simulink model "Tractive_Motor_Ring_Single_Motor"  (R2020a)
settings: Solver=FixedStepDiscrete  StartTime=0.0  StopTime=10.0  FixedStep=Ts  RelTol=1e-3  EnableMultiTasking=on
PostLoadFcn:
  | , if any(exist('dsrtsu_mdlpostloadfcn', 'file') ~= 0), dsrtsu_mdlpostloadfcn('Execute', bdroot); end,
InitFcn:
  | , if any(exist('rtifpga_mdlclblib', 'file') ~= 0), rtifpga_mdlclblib('Init', bdroot); end,
undefined symbols (not defined in the file): DiscIntNeverNeededParam, magnitude, TMR
libraries: simulink x3
settings Model: DSRTSU_INTERNAL_RTI_VER=560  DSRTSU_INTERNAL_RTI_TYPE=rti1401  RTICANMMDATA=struct('GeneralSetupData',struct('modelroot','C:\Users\harjo\Git\MACFormulaGit\MicroAutobox\rings\Tractive_Motor_Ring\Tractive_Motor_Ring_Single_Motor','generalsettings',struct('filesettings',struct('destfolder',struct('Name','RTICANMM_FILES','Check',1),'buildfolder',struct('Name','.','Check',1),'AbsDestfolder',struct('Name','C:\Users\harjo\Git\MACFormulaGit\MicroAutobox\rings\Tractive_Motor_Ring\Tractive_Motor_Ring_Single_Motor\RTICANMM_FILES'),'AbsBuildfolder',struct('Name','C:\Users\harjo\Git\MACFormulaGit\MicroAutobox\rings\Tractive_Motor_Ring\Tractive_Motor_Ring_Single_Motor'))),'options',struct('addpaths',1,'rmpaths',1,'addtrcexclusion',true,'cannavigator',struct('checkmonitoring',0),'show_usrtrc',0,'use_usrtrc',0),'advanced',struct('options',ones(1,100)),'MPSetup',{{}},'RTI',struct('Type','RTI1401','Ver','7.14','Date','02-May-2020'),'modelname','Tractive_Motor_Ring_Single_Motor','block','Tractive_Motor_Ring_Single_Motor'))  DSRTSU_INTERNAL_RTIFPGA=160  Creator=Harjot  LastModifiedBy=Harjot
settings DebuggingCC: SFUnexpectedBacktrackingDiag=warning  SFNoUnconditionalDefaultTransitionDiag=warning  SFExecutionAtInitializationDiag=none  ArithmeticOperatorsInVariantConditions=warning
settings HardwareCC: ProdBitPerPointer=32  ProdBitPerSizeT=32  ProdBitPerPtrDiffT=32  ProdLargestAtomicInteger=Integer  ProdEndianess=BigEndian  ProdWordSize=32  ProdHWDeviceType=Custom Processor->Custom  TargetIntDivRoundTo=Zero  TargetEndianess=BigEndian  TargetHWDeviceType=Custom Processor->Custom
settings SFSimCC: SimUseLocalCustomCode=off  MATLABDynamicMemAlloc=off  CustomCodeUndefinedFunction=UseInterfaceOnly
settings RTWCC: Description=dSPACE DS1401 Hardware Platform  SystemTargetFile=rti1401.tlc  MakeCommand=make_rti  TemplateMakefile=rti1401.tmf  RTWUseLocalCustomCode=off
settings CodeAppCC: StateflowObjectComments=on
settings STFCustomTargetCC: UtilityFuncGeneration=Shared location  ParMdlRefBuildCompliant=on  SystemTargetFile=rti1401.tlc
settings GRTTargetCC: TargetLangStandard=C89/C90 (ANSI)  UtilityFuncGeneration=Shared location  CompOptLevelCompliant=off  ConcurrentExecutionCompliant=off  CombineOutputUpdateFcns=off  MatFileLogging=off  CPPClassGenCompliant=off  UseToolchainInfoCompliant=off
settings ConfigComp: CovMetricSettings=dw  CovHtmlReporting=on  CovSaveCumulativeToWorkspaceVar=on  CovSaveSingleToWorkspaceVar=on  CovExternalEMLEnable=off

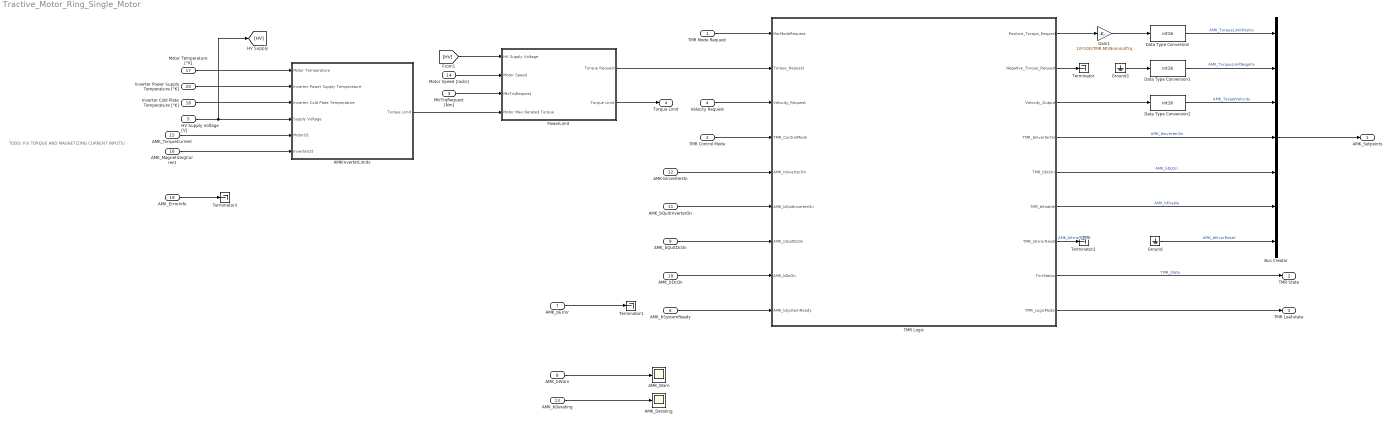
== system Tractive_Motor_Ring_Single_Motor ==
  note: TODO: FIX TORQUE AND MAGNETIZING CURRENT INPUTS!
  TMR Mode Request : Inport
  TMR Control Mode : Inport  Port=2
  MtrTrqRequest [Nm] : Inport  Port=3
  Velocity Request : Inport  Port=4
  HV Supply Voltage [V] : Inport  Port=5
  AMK_bSystemReady : Inport  Port=6  OutDataTypeStr=boolean  Interpolate=off  LockScale=on
  AMK_bError : Inport  Port=7  OutDataTypeStr=boolean  Interpolate=off  LockScale=on
  AMK_bWarn : Inport  Port=8  OutDataTypeStr=boolean  Interpolate=off
  AMK_bQuitDcOn : Inport  Port=9  OutDataTypeStr=boolean  Interpolate=off  LockScale=on
  AMK_bDcOn : Inport  Port=10  OutDataTypeStr=boolean  Interpolate=off  LockScale=on
  AMK_bQuitInverterOn : Inport  Port=11  OutDataTypeStr=boolean  LockScale=on
  AMK-bInverterOn : Inport  Port=12  OutDataTypeStr=boolean  Interpolate=off  LockScale=on
  AMK_bDerating : Inport  Port=13  OutDataTypeStr=boolean  Interpolate=off
  Motor Speed [rad/s] : Inport  Port=14
  AMK_TorqueCurrent : Inport  Port=15
  AMK_MagnetizingCurrent : Inport  Port=16
  Motor Temperature [°K] : Inport  Port=17  OutDataTypeStr=double
  Inverter Cold Plate Temperature [°K] : Inport  Port=18  OutDataTypeStr=double
  AMK_ErrorInfo : Inport  Port=19  OutDataTypeStr=double
  Inverter Power Supply Temperature [°K] : Inport  Port=20  OutDataTypeStr=double
  AMKInverterLimits : Subsystem
  AMK_Derating : Scope
  AMK_Warn : Scope
  Bus Creator : BusCreator  Inputs=7  OutDataTypeStr=Bus: AmkSetpoints  NonVirtualBus=on
      settings: InheritFromInputs=off
  Data Type Conversion : DataTypeConversion  OutDataTypeStr=int16
  Data Type Conversion1 : DataTypeConversion  OutDataTypeStr=int16
  Data Type Conversion2 : DataTypeConversion  OutDataTypeStr=int16
  Gain1 : Gain  Gain=10*100/TMR.MtrNominalTrq
  Ground : Ground
  Ground1 : Ground
  PowerLimit : Subsystem
  TMR Logic : Stateflow chart  TreatAsAtomicUnit=on
  Terminator{,1..3} (4 alike) : Terminator
  AMK_Setpoints : Outport  OutDataTypeStr=Bus: AmkSetpoints  VectorParamsAs1DForOutWhenUnconnected=off
  TMR State : Outport  Port=2  VectorParamsAs1DForOutWhenUnconnected=off
  TMR Leaf-state : Outport  Port=3  VectorParamsAs1DForOutWhenUnconnected=off
  Torque Limit : Outport  Port=4  VectorParamsAs1DForOutWhenUnconnected=off
  wires:
  TMR Logic/4(TMR_bInverterOn) -> Bus Creator/4  "AMK_bInverterOn"
  TMR Logic/6(TMR_bEnable) -> Bus Creator/6  "AMK_bEnable"
  TMR Logic/5(TMR_bDcOn) -> Bus Creator/5  "AMK_bDcOn"
  AMK_ErrorInfo/1 -> Terminator3/1
  AMK_bDerating/1 -> AMK_Derating/1
  AMK_bWarn/1 -> AMK_Warn/1
  Velocity Request/1 -> TMR Logic/3(Velocity_Request)
  AMK_bSystemReady/1 -> TMR Logic/9(AMK_bSystemReady)
  AMK_bQuitInverterOn/1 -> TMR Logic/6(AMK_bQuitInverterOn)
  Bus Creator/1 -> AMK_Setpoints/1
  TMR Logic/1(Positive_Torque_Request) -> Gain1/1
  TMR Control Mode/1 -> TMR Logic/4(TMR_ControlMode)
  TMR Logic/9(TMR_LogicMode) -> TMR Leaf-state/1
  Ground/1 -> Bus Creator/7  "AMK_bErrorReset"
  AMK_bQuitDcOn/1 -> TMR Logic/7(AMK_bQuitDcOn)
  AMK-bInverterOn/1 -> TMR Logic/5(AMK_bInverterOn)
  AMK_bDcOn/1 -> TMR Logic/8(AMK_bDcOn)
  TMR Logic/8(TmrStatus) -> TMR State/1  "TMR_State"
  TMR Mode Request/1 -> TMR Logic/1(MsrModeRequest)
  Data Type Conversion/1 -> Bus Creator/1  "AMK_TorqueLimitPositiv"
  Data Type Conversion1/1 -> Bus Creator/2  "AMK_TorqueLimitNegativ"
  Data Type Conversion2/1 -> Bus Creator/3  "AMK_TargetVelocity"
  TMR Logic/3(Velocity_Output) -> Data Type Conversion2/1
  Gain1/1 -> Data Type Conversion/1
  Ground1/1 -> Data Type Conversion1/1
  TMR Logic/2(Negative_Torque_Request) -> Terminator/1
  AMK_bError/1 -> Terminator1/1
  TMR Logic/7(TMR_bErrorReset) -> Terminator2/1  "AMK_bErrorReset"
  AMKInverterLimits/1(Torque Limit) -> PowerLimit/4(Motor Max Derated Torque)
  AMK_MagnetizingCurrent/1 -> AMKInverterLimits/6(InverterI2t)
  AMK_TorqueCurrent/1 -> AMKInverterLimits/5(MotorI2t)
  [HV] -> PowerLimit/1(HV Supply Voltage)
  HV Supply Voltage [V]/1 -> [HV], AMKInverterLimits/4(Supply Voltage)
  Inverter Cold Plate Temperature [°K]/1 -> AMKInverterLimits/3(Inverter Cold Plate Temperature)
  Inverter Power Supply Temperature [°K]/1 -> AMKInverterLimits/2(Inverter Power Supply Temperature)
  Motor Temperature [°K]/1 -> AMKInverterLimits/1(Motor Temperature)
  MtrTrqRequest [Nm]/1 -> PowerLimit/3(MtrTrqRequest)
  PowerLimit/1(Torque Request) -> TMR Logic/2(Torque_Request)
  PowerLimit/2(Torque Limit) -> Torque Limit/1
  Motor Speed [rad/s]/1 -> PowerLimit/2(Motor Speed)

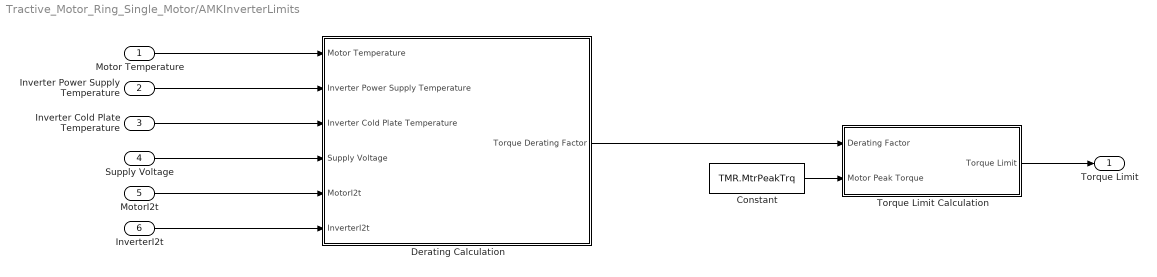
== system Tractive_Motor_Ring_Single_Motor/AMKInverterLimits ==
  Motor Temperature : Inport
  Inverter Power Supply Temperature : Inport  Port=2
  Inverter Cold Plate Temperature : Inport  Port=3
  Supply Voltage : Inport  Port=4
  MotorI2t : Inport  Port=5
  InverterI2t : Inport  Port=6
  Constant : Constant  Value=TMR.MtrPeakTrq
  Derating Calculation : Subsystem
  Torque Limit Calculation : Subsystem
  Torque Limit : Outport  VectorParamsAs1DForOutWhenUnconnected=off
  wires:
  Torque Limit Calculation/1(Torque Limit) -> Torque Limit/1
  InverterI2t/1 -> Derating Calculation/6(InverterI2t)
  Inverter Power Supply Temperature/1 -> Derating Calculation/2(Inverter Power Supply Temperature)
  Constant/1 -> Torque Limit Calculation/2(Motor Peak Torque)
  Motor Temperature/1 -> Derating Calculation/1(Motor Temperature)
  Derating Calculation/1(Torque Derating Factor) -> Torque Limit Calculation/1(Derating Factor)
  Inverter Cold Plate Temperature/1 -> Derating Calculation/3(Inverter Cold Plate Temperature)
  MotorI2t/1 -> Derating Calculation/5(MotorI2t)
  Supply Voltage/1 -> Derating Calculation/4(Supply Voltage)

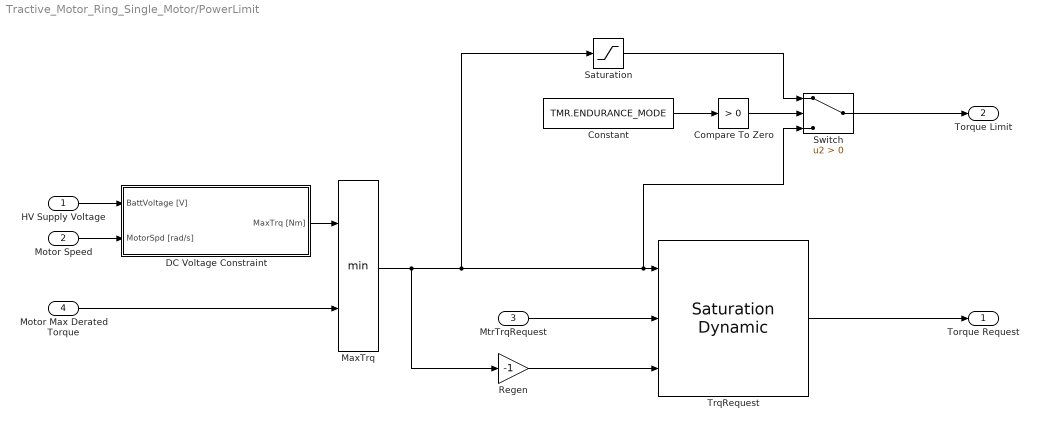
== system Tractive_Motor_Ring_Single_Motor/PowerLimit ==
  HV Supply Voltage : Inport
  Motor Speed : Inport  Port=2
  MtrTrqRequest : Inport  Port=3
  Motor Max Derated Torque : Inport  Port=4
  Compare To Zero : simulink/Logic and Bit Operations/Compare To Zero  relop=>  OutDataTypeStr=boolean
  Constant : Constant  Value=TMR.ENDURANCE_MODE
  DC Voltage Constraint : Subsystem
  MaxTrq : MinMax  Inputs=2
  Regen : Gain  Gain=-1
  Saturation : Saturate  UpperLimit=TMR.MtrNominalTrq  LowerLimit=0
  Switch : Switch  Criteria=u2 > Threshold
  TrqRequest : simulink/Discontinuities/Saturation Dynamic  OutMin=[]  OutMax=[]  OutDataTypeStr=Inherit: Same as second input  OutDataType=fixdt(1, 16)  OutScaling=2^-10  DoSatur=off
  Torque Request : Outport  VectorParamsAs1DForOutWhenUnconnected=off
  Torque Limit : Outport  Port=2  VectorParamsAs1DForOutWhenUnconnected=off
  wires:
  Saturation/1 -> Switch/1
  Switch/1 -> Torque Limit/1
  Compare To Zero/1 -> Switch/2
  Constant/1 -> Compare To Zero/1
  Regen/1 -> TrqRequest/3
  HV Supply Voltage/1 -> DC Voltage Constraint/1(BattVoltage [V])
  DC Voltage Constraint/1(MaxTrq [Nm]) -> MaxTrq/1
  MaxTrq/1 -> TrqRequest/1, Switch/3, Saturation/1, Regen/1
  Motor Speed/1 -> DC Voltage Constraint/2(MotorSpd [rad/s])
  TrqRequest/1 -> Torque Request/1
  Motor Max Derated Torque/1 -> MaxTrq/2
  MtrTrqRequest/1 -> TrqRequest/2

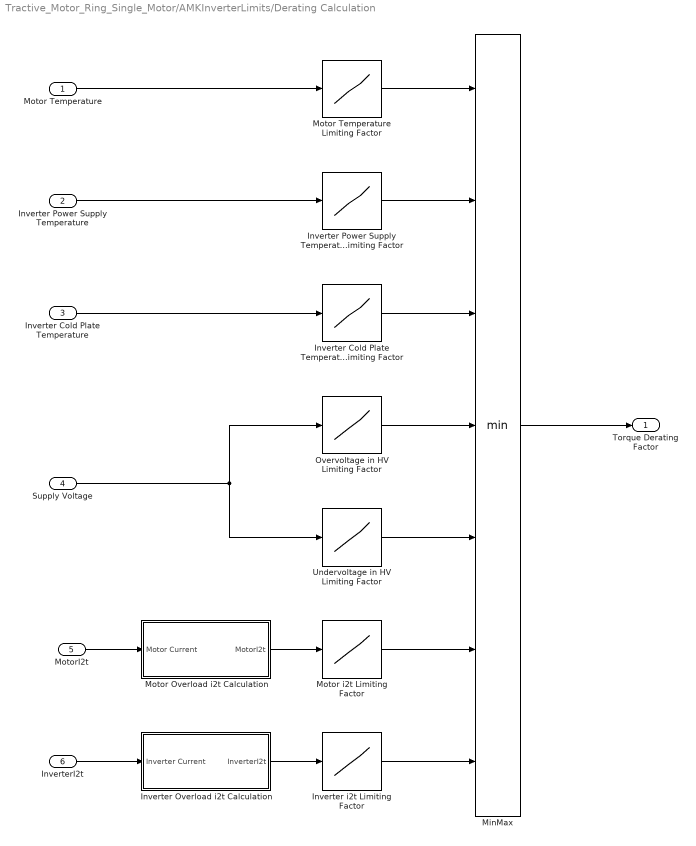
== system Tractive_Motor_Ring_Single_Motor/AMKInverterLimits/Derating Calculation ==
  Motor Temperature : Inport
  Inverter Power Supply Temperature : Inport  Port=2
  Inverter Cold Plate Temperature : Inport  Port=3
  Supply Voltage : Inport  Port=4
  MotorI2t : Inport  Port=5
  InverterI2t : Inport  Port=6
  Inverter Cold Plate Temperature Limiting Factor : Lookup_n-D  NumberOfTableDimensions=1  BreakpointsForDimension1=[TMR.ColdPlateTempFullTrq, TMR.ColdPlateTempNoTrq]  Table=[1,0]  ExtrapMethod=Clip  InternalRulePriority=Speed  RndMeth=Simplest  InputSameDT=on
  Inverter Overload i2t Calculation : Subsystem
  Inverter Power Supply Temperature Limiting Factor : Lookup_n-D  NumberOfTableDimensions=1  BreakpointsForDimension1=[TMR.PwrSpplyTempFullTrq, TMR.PwrSpplyTempNoTrq]  Table=[1,0]  ExtrapMethod=Clip  InternalRulePriority=Speed  RndMeth=Simplest  InputSameDT=on
  Inverter i2t Limiting Factor : Lookup_n-D  NumberOfTableDimensions=1  BreakpointsForDimension1=[TMR.InvCurrOverloadThreshold*TMR.InvI2t, TMR.InvI2t]  Table=[1,0]  ExtrapMethod=Clip  InternalRulePriority=Speed  RndMeth=Simplest  InputSameDT=on
  MinMax : MinMax  Inputs=7
  Motor Overload i2t Calculation : Subsystem
  Motor Temperature Limiting Factor : Lookup_n-D  NumberOfTableDimensions=1  BreakpointsForDimension1=[TMR.MtrTempFullTrq, TMR.MtrTempNoTrq]  Table=[1,0]  ExtrapMethod=Clip  InternalRulePriority=Speed  RndMeth=Simplest  InputSameDT=on
  Motor i2t Limiting Factor : Lookup_n-D  NumberOfTableDimensions=1  BreakpointsForDimension1="[TMR.MtrCurrOverloadThreshold*TMR.MtrI2t,  TMR.MtrI2t]"  Table=[1,0]  ExtrapMethod=Clip  InternalRulePriority=Speed  RndMeth=Simplest  InputSameDT=on
  Overvoltage in HV Limiting Factor : Lookup_n-D  NumberOfTableDimensions=1  BreakpointsForDimension1=[TMR.HighBatteryVolt, TMR.MaxBatteryVolt]  Table=[1,0]  ExtrapMethod=Clip  InternalRulePriority=Speed  RndMeth=Simplest  InputSameDT=on
  Undervoltage in HV Limiting Factor : Lookup_n-D  NumberOfTableDimensions=1  BreakpointsForDimension1=[TMR.MinBatteryVolt, TMR.LowBatteryVolt]  Table=[0,1]  ExtrapMethod=Clip  InternalRulePriority=Speed  RndMeth=Simplest  InputSameDT=on
  Torque Derating Factor : Outport  VectorParamsAs1DForOutWhenUnconnected=off
  wires:
  Motor i2t Limiting Factor/1 -> MinMax/6
  Inverter i2t Limiting Factor/1 -> MinMax/7
  InverterI2t/1 -> Inverter Overload i2t Calculation/1(Inverter Current)
  Undervoltage in HV Limiting Factor/1 -> MinMax/5
  Inverter Power Supply Temperature Limiting Factor/1 -> MinMax/2
  Motor Temperature Limiting Factor/1 -> MinMax/1
  Overvoltage in HV Limiting Factor/1 -> MinMax/4
  Motor Temperature/1 -> Motor Temperature Limiting Factor/1
  Inverter Cold Plate Temperature Limiting Factor/1 -> MinMax/3
  Inverter Cold Plate Temperature/1 -> Inverter Cold Plate Temperature Limiting Factor/1
  Inverter Power Supply Temperature/1 -> Inverter Power Supply Temperature Limiting Factor/1
  MotorI2t/1 -> Motor Overload i2t Calculation/1(Motor Current)
  Motor Overload i2t Calculation/1(MotorI2t) -> Motor i2t Limiting Factor/1
  Supply Voltage/1 -> Undervoltage in HV Limiting Factor/1, Overvoltage in HV Limiting Factor/1
  Inverter Overload i2t Calculation/1(InverterI2t) -> Inverter i2t Limiting Factor/1
  MinMax/1 -> Torque Derating Factor/1

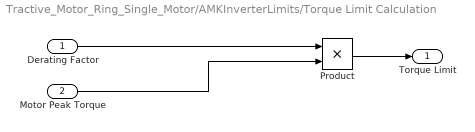
== system Tractive_Motor_Ring_Single_Motor/AMKInverterLimits/Torque Limit Calculation ==
  Derating Factor : Inport
  Motor Peak Torque : Inport  Port=2
  Product : Product
  Torque Limit : Outport  VectorParamsAs1DForOutWhenUnconnected=off
  wires:
  Product/1 -> Torque Limit/1
  Derating Factor/1 -> Product/1
  Motor Peak Torque/1 -> Product/2

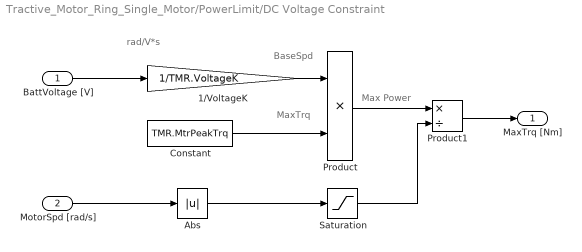
== system Tractive_Motor_Ring_Single_Motor/PowerLimit/DC Voltage Constraint ==
  note: Max Power
  note: MaxTrq
  note: BaseSpd
  note: rad/V*s
  BattVoltage [V] : Inport
  MotorSpd [rad/s] : Inport  Port=2
  1/VoltageK : Gain  Gain=1/TMR.VoltageK
  Abs : Abs
  Constant : Constant  Value=TMR.MtrPeakTrq
  Product : Product
  Product1 : Product  Inputs=*/
  Saturation : Saturate  UpperLimit=10000  LowerLimit=TMR.MinMtrSpd
  MaxTrq [Nm] : Outport  VectorParamsAs1DForOutWhenUnconnected=off
  wires:
  Saturation/1 -> Product1/2
  Product/1 -> Product1/1
  BattVoltage [V]/1 -> 1/VoltageK/1
  Constant/1 -> Product/2
  Product1/1 -> MaxTrq [Nm]/1
  MotorSpd [rad/s]/1 -> Abs/1
  1/VoltageK/1 -> Product/1
  Abs/1 -> Saturation/1

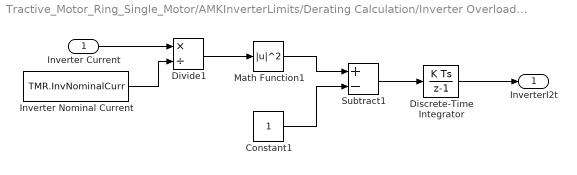
== system Tractive_Motor_Ring_Single_Motor/AMKInverterLimits/Derating Calculation/Inverter Overload i2t Calculation ==
  Inverter Current : Inport
  Constant1 : Constant
  Discrete-Time Integrator : DiscreteIntegrator  SampleTime=-1  ICPrevOutput=DiscIntNeverNeededParam  ICPrevScaledInput=DiscIntNeverNeededParam
  Divide1 : Product  Inputs=*/
  Inverter Nominal Current : Constant  Value=TMR.InvNominalCurr
  Math Function1 : Math  Operator=magnitude^2  SignedPower=on  SaturateOnIntegerOverflow=on
  Subtract1 : Sum  Inputs=+-
  InverterI2t : Outport  VectorParamsAs1DForOutWhenUnconnected=off
  wires:
  Subtract1/1 -> Discrete-Time Integrator/1
  Constant1/1 -> Subtract1/2
  Inverter Nominal Current/1 -> Divide1/2
  Discrete-Time Integrator/1 -> InverterI2t/1
  Inverter Current/1 -> Divide1/1
  Divide1/1 -> Math Function1/1
  Math Function1/1 -> Subtract1/1

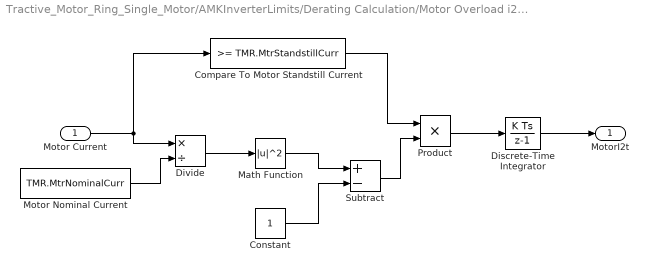
== system Tractive_Motor_Ring_Single_Motor/AMKInverterLimits/Derating Calculation/Motor Overload i2t Calculation ==
  Motor Current : Inport
  Compare To Motor Standstill Current : simulink/Logic and Bit Operations/Compare To Constant  relop=>=  const=TMR.MtrStandstillCurr  OutDataTypeStr=boolean
  Constant : Constant
  Discrete-Time Integrator : DiscreteIntegrator  SampleTime=-1  ICPrevOutput=DiscIntNeverNeededParam  ICPrevScaledInput=DiscIntNeverNeededParam
  Divide : Product  Inputs=*/
  Math Function : Math  Operator=magnitude^2  SignedPower=on  SaturateOnIntegerOverflow=on
  Motor Nominal Current : Constant  Value=TMR.MtrNominalCurr
  Product : Product
  Subtract : Sum  Inputs=+-
  MotorI2t : Outport  VectorParamsAs1DForOutWhenUnconnected=off
  wires:
  Motor Current/1 -> Divide/1, Compare To Motor Standstill Current/1
  Divide/1 -> Math Function/1
  Math Function/1 -> Subtract/1
  Subtract/1 -> Product/2
  Compare To Motor Standstill Current/1 -> Product/1
  Motor Nominal Current/1 -> Divide/2
  Product/1 -> Discrete-Time Integrator/1
  Constant/1 -> Subtract/2
  Discrete-Time Integrator/1 -> MotorI2t/1

== stateflow chart Tractive_Motor_Ring_Single_Motor/TMR Logic ==
  state NORMAL_OPERATION
    (history)
    state OFF
      entry:
      TmrStatus = RING_STATUS.OFF;
      Positive_Torque_Request = 0;
      Negative_Torque_Request = 0;
      Velocity_Output = 0;
      TMR_bInverterOn = false;
      TMR_bDcOn = false;
      TMR_bEnable = false;
      TMR_bErrorReset = false;
    state SHUTDOWN
      entry:
      TmrStatus = RING_STATUS.SHUTDOWN_IN_PROGRESS_HV;
      state RequirementsShutDown
        entry:
        Positive_Torque_Request = 0;
        Negative_Torque_Request = 0;
        Velocity_Output = 0;
      state ResetX140BE2
        entry:
        %Reset X140BE2
      state ResetInverterOn
        entry:
        TMR_bInverterOn = false;
      state ResetEnable
        entry:
        TMR_bEnable = false;
      state ResetX140BE1
        entry:
        %Reset X140BE1
      state ShutDown
        entry:
        TmrStatus = RING_STATUS.SHUTDOWN_COMPLETE_HV;
      state CheckQuitDcON1
        entry:
      state ResetX15EF1EF2
        entry:
        %Reset X15EF1/EF2
      state HV_Deactivation
        entry:
        TMR_bDcOn = false;
      (default) -> RequirementsShutDown
      RequirementsShutDown -> ResetX140BE2
      ResetEnable -> ResetX140BE1 : [~AMK_bQuitDcOn]
      ResetX140BE2 -> ResetInverterOn
      ResetInverterOn -> ResetEnable : [~AMK_bInverterOn]
      ResetX140BE1 -> ResetX15EF1EF2
      CheckQuitDcON1 -> ShutDown : [~AMK_bQuitDcOn]
      HV_Deactivation -> CheckQuitDcON1 : [~AMK_bDcOn]
      ResetX15EF1EF2 -> HV_Deactivation
    state OPERATIONAL
      state STARTUP_LV
        entry:
        TmrStatus = RING_STATUS.STARTUP_IN_PROGRESS_LV;
        state AMK_CHECK
          entry:
        state AMK_ONLINE
          entry:
          TmrStatus = RING_STATUS.STARTUP_COMPLETE_LV;
        (default) -> AMK_CHECK
        AMK_CHECK -> AMK_ONLINE : [AMK_bSystemReady]
      state RUNNING
        entry:
        TmrStatus = RING_STATUS.RUNNING;
        state ControlModeOff
          during:
          Positive_Torque_Request = 0;
          Negative_Torque_Request = 0;
          Velocity_Output = 0;
        state SetpointSettingsTorqueControl
          state ForwardAccelSetpointSettingsTorqueControl
            during:
            Velocity_Output = 30000;
            Positive_Torque_Request = Torque_Request;
            Negative_Torque_Request = 0;
          state BrakingSetpointSettingsTorqueControl
            during:
            Velocity_Output = 0; % 750 rpm, = 5km/h
            Positive_Torque_Request = 0;
            Negative_Torque_Request = Torque_Request
          (default) -> (junction 182)
          (junction 182) -> ForwardAccelSetpointSettingsTorqueControl [order 1] : [Torque_Request >= 0]
          (junction 182) -> BrakingSetpointSettingsTorqueControl [order 2]
          ForwardAccelSetpointSettingsTorqueControl -> BrakingSetpointSettingsTorqueControl : [Torque_Request < 0]
          BrakingSetpointSettingsTorqueControl -> ForwardAccelSetpointSettingsTorqueControl : [Torque_Request >= 0]
        state SetpointSettingsSpeedControl
          during:
          Velocity_Output = Velocity_Request;
          Positive_Torque_Request = Torque_Request;
          Negative_Torque_Request = -1*Torque_Request;
        (default) -> ControlModeOff
        ControlModeOff -> SetpointSettingsTorqueControl [order 1] : [TMR_ControlMode == TMR.CONTROL_MODE.TORQUE_CONTROL]
        ControlModeOff -> SetpointSettingsSpeedControl [order 2] : [TMR_ControlMode == TMR.CONTROL_MODE.SPEED_CONTROL]
        SetpointSettingsSpeedControl -> ControlModeOff [order 2] : [TMR_ControlMode == TMR.CONTROL_MODE.OFF]
        SetpointSettingsTorqueControl -> ControlModeOff [order 2] : [TMR_ControlMode == TMR.CONTROL_MODE.OFF]
        SetpointSettingsSpeedControl -> SetpointSettingsTorqueControl [order 1] : [TMR_ControlMode == TMR.CONTROL_MODE.TORQUE_CONTROL]
        SetpointSettingsTorqueControl -> SetpointSettingsSpeedControl [order 1] : [TMR_ControlMode == TMR.CONTROL_MODE.SPEED_CONTROL]
      state STARTUP_HV
        entry:
        TmrStatus = RING_STATUS.STARTUP_IN_PROGRESS_HV;
        state Requirements
          entry:
          Positive_Torque_Request = 0;
          Negative_Torque_Request = 0;
          Velocity_Output = 0;
        state StartingStartUpSequence
        state CheckQuitDcON
          entry:
        state SetX15EF1EF2
          entry:
          %Set X15EF1/EF2
        state HV_Activation
          entry:
          TMR_bDcOn = true;
        state StartUpPass
          entry:
          TmrStatus = RING_STATUS.STARTUP_COMPLETE_HV;
        state SetX140BE2
          entry:
          %Set X140BE2
        state CheckQuitInverterOn
          entry:
        state SetInverterOn
          entry:
          TMR_bInverterOn = true;
        state SetEnable
          entry:
          TMR_bEnable = true;
        state SetX140BE1
          entry:
          %Set X140BE1
        (default) -> StartingStartUpSequence
        Requirements -> SetX15EF1EF2
        CheckQuitDcON -> Requirements : [AMK_bQuitDcOn]
        HV_Activation -> CheckQuitDcON : [AMK_bDcOn]
        StartingStartUpSequence -> HV_Activation
        SetX15EF1EF2 -> SetX140BE1
        SetEnable -> SetInverterOn
        SetX140BE1 -> SetEnable
        SetInverterOn -> CheckQuitInverterOn : [AMK_bInverterOn]
        SetX140BE2 -> StartUpPass
        CheckQuitInverterOn -> SetX140BE2 : [AMK_bQuitInverterOn]
      (default) -> STARTUP_LV
      STARTUP_LV -> STARTUP_HV : [MsrModeRequest == MSR_REQUEST.STARTUP_HV &&...
          |  TmrStatus == RING_STATUS.STARTUP_COMPLETE_LV]
      STARTUP_HV -> RUNNING : [MsrModeRequest == MSR_REQUEST.RUNNING &&...
          | TmrStatus == RING_STATUS.STARTUP_COMPLETE_HV]
    (default) -> OFF
    OPERATIONAL -> SHUTDOWN : [MsrModeRequest == MSR_REQUEST.SHUTDOWN_HV]
    OFF -> OPERATIONAL : [MsrModeRequest == MSR_REQUEST.STARTUP_LV]
  (default) -> NORMAL_OPERATION
  data: MsrModeRequest input Enum: MSR_REQUEST; Torque_Request input; Positive_Torque_Request output double; Negative_Torque_Request output double; Velocity_Output output double; TMR_bInverterOn output boolean; TMR_bDcOn output boolean; TMR_bEnable output boolean; TMR_bErrorReset output boolean; TmrStatus output Enum: RING_STATUS; Velocity_Request input; TMR_ControlMode input; AMK_bInverterOn input boolean; AMK_bQuitInverterOn input boolean; AMK_bQuitDcOn input boolean; AMK_bDcOn input boolean; AMK_bSystemReady input boolean; TMR parameter; TMR_LogicMode output Enum: TMR_LogicModeType
